simulink model "first_order_open_closed_loop"  (R2023a)
settings: Solver=VariableStepAuto  StartTime=0.0  StopTime=10.0  MaxStep=1e-6
settings Model: Creator=mazen  LastModifiedBy=mazen

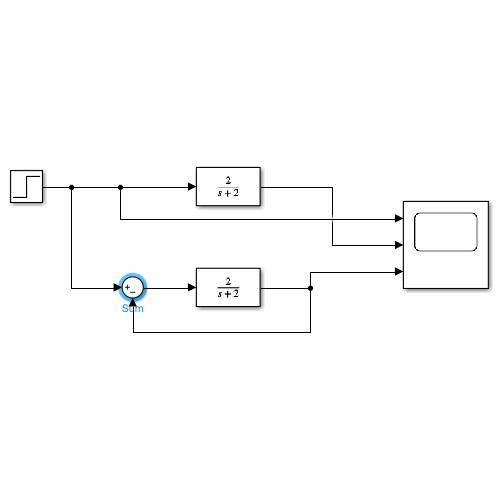
[thumbnail: Simulink's stored preview of the top-level diagram]
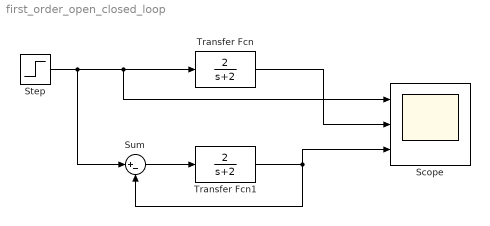
== system first_order_open_closed_loop ==
  Scope : Scope  NumInputPorts=3
  Step : Step  SampleTime=0
  Sum : Sum  Inputs=|+-
  Transfer Fcn : TransferFcn  Numerator=[2]  Denominator=[1 2]
  Transfer Fcn1 : TransferFcn  Numerator=[2]  Denominator=[1 2]
  wires:
  Transfer Fcn/1 -> Scope/2
  Step/1 -> Sum/1, Transfer Fcn/1, Scope/1
  Sum/1 -> Transfer Fcn1/1
  Transfer Fcn1/1 -> Sum/2, Scope/3
